simulink model "untitled"  (R2024b)
settings: Solver=VariableStepAuto  StartTime=0.0  StopTime=10.0  RelTol=1e-3
values from neighbouring files (symbols this model uses):
  pitch_force = [0         0         0         0    1.0000         0]    [constants.m]
  roll_force = [0         0         0    0.5000         0         0]    [constants.m]
  x_force = [0.4100         0         0         0         0         0]    [constants.m]    (also in init2.m = [0.410000000000000	0	0	0	0	0])
  y_force = [0    0.5000         0         0         0         0]    [constants.m]    (also in init2.m = [0	0.500000000000000	0	0	0	0])
  yaw_force = [0         0         0         0         0    0.5000]    [constants.m]
  z_force = [0         0    1.2500         0         0         0]    [constants.m]
settings Model: Creator=vinso  LastModifiedBy=vinso

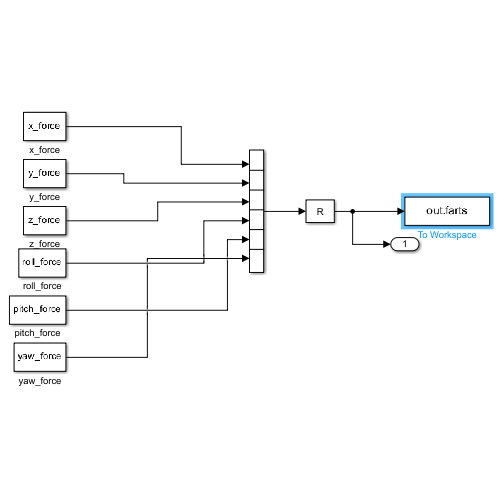
[thumbnail: Simulink's stored preview of the top-level diagram]
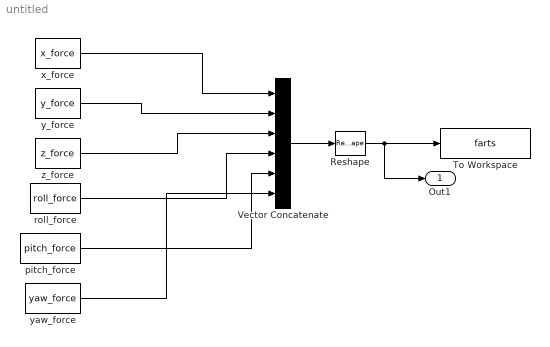
== system untitled ==
  Reshape : Reshape  OutputDimensionality=Customize  OutputDimensions=[6,6]
  To Workspace : ToWorkspace  VariableName=farts  SampleTime=-1
      settings: Save2DSignal=2-D array (concatenate along first dimension)
  Vector Concatenate : Concatenate  NumInputs=6
  pitch_force : Constant  Value=pitch_force  VectorParams1D=off
  roll_force : Constant  Value=roll_force  VectorParams1D=off
  x_force : Constant  Value=x_force  VectorParams1D=off
  y_force : Constant  Value=y_force  VectorParams1D=off
  yaw_force : Constant  Value=yaw_force  VectorParams1D=off
  z_force : Constant  Value=z_force  VectorParams1D=off
  Out1 : Outport
  wires:
  y_force/1 -> Vector Concatenate/2
  z_force/1 -> Vector Concatenate/3
  roll_force/1 -> Vector Concatenate/4
  pitch_force/1 -> Vector Concatenate/5
  Vector Concatenate/1 -> Reshape/1
  yaw_force/1 -> Vector Concatenate/6
  x_force/1 -> Vector Concatenate/1
  Reshape/1 -> Out1/1, To Workspace/1
